simulink model "Joint_data_model"  (R2012b)
settings: Solver=ode1  StartTime=0.0  StopTime=10  FixedStep=0.002  RelTol=1e-3
settings Model: ExtModeTrigDuration=5000  Creator=crbonney  LastModifiedBy=crbonney
settings SolverCC: PositivePriorityOrder=on
settings RTWCC: SystemTargetFile=quarc_win64.tlc  TemplateMakefile=quarc_default_tmf  Description=QUARC Win64 Target  ProcessScript=quarc_win64_make_rtw_hook
settings STFCustomTargetCC: TargetPreCompLibLocation=C:\PROGRA~3\QUARC\lib\2012b\win64\release  CodeReplacementLibrary=ANSI_C  GeneratePreprocessorConditionals=Disable all  CombineOutputUpdateFcns=on  GRTInterface=off  SystemTargetFile=quarc_win64.tlc
settings GRTTargetCC: TargetPreCompLibLocation=C:\PROGRA~3\QUARC\lib\2012b\win64\release  ParMdlRefBuildCompliant=off  CompOptLevelCompliant=off  ConcurrentExecutionCompliant=off  MatFileLogging=off  ExtMode=on  ExtModeMexFile=quarc_comm

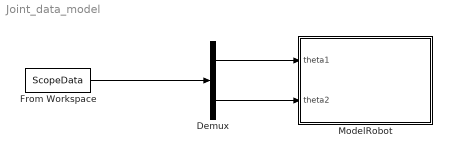
== system Joint_data_model ==
  Demux : Demux  Outputs=2
  From Workspace : FromWorkspace  VariableName=ScopeData  SampleTime=0
  ModelRobot : MATLAB Function  TreatAsAtomicUnit=on
  wires:
  From Workspace/1 -> Demux/1
  Demux/1 -> ModelRobot/1(theta1)
  Demux/2 -> ModelRobot/2(theta2)

== matlab function Joint_data_model/ModelRobot ==
  data: theta1 input; theta2 input
function ModelRobot (theta1, theta2)
    frame0_links = ...
        [0  0;...  %X
         0  0;...  %Y
         0 -15];   %Z

    frame1_links = ...
        [0  0  0  0 0;... %X
         0  0  6  6 8;... %Y
         0 -1 -1  0 0];   %Z

    frame2_links = ...
        [0   0;... %X
         0  12;... %Y
         0   0];   %Z

    rho = sqrt(8^2+12^2);
    phi_max = atan(12/8);

    f1 = TransformPoints(TRANS0_1(theta1),frame1_links);
    f2 = TransformPoints(TRANS0_1(theta1),TransformPoints(TRANS1_2(theta2),frame2_links));


    plot3(frame0_links(1,:),frame0_links(2,:), frame0_links(3,:),'bs-','LineWidth',3);
    axis([-15 15 -15 15 -15 15]);
    grid on
    hold on
    xlabel('x');
    ylabel('y');
    zlabel('z');
    plot3(f1(1,:),f1(2,:), f1(3,:),'rs-','LineWidth',3);
    plot3(f2(1,:),f2(2,:), f2(3,:),'go-', 'MarkerFaceColor', 'c', 'MarkerSize',5,'LineWidth',3);
    plot3(f2(1,end),f2(2,end), f2(3,end),'go-', 'MarkerFaceColor', 'c', 'MarkerSize',5,'LineWidth',3);
    axis([-15 15 -15 15 -15 15]);
    WorkEnvelope2(rho, phi_max);
    hold off
end
